simulink model "q4conversor"  (R2023b)
settings: Solver=VariableStepAuto  StartTime=0.0  StopTime=4e-3  RelTol=1e-3
values from neighbouring files (symbols this model uses):
  C = 100e-6    (= 0.0001)    [q4.m]
  Gatr = zpk(Gatr)    [q4.m]
  Gavan = zpk(Gavan)    [q4.m]
  Kc = 198    [q4.m]
  Kd = npid(1)    [q4.m]
  Ki = npid(3)    [q4.m]
  Kp = npid(2)    [q4.m]
  L = 100e-6    (= 0.0001)    [q4.m]
  Rc = 0.5    [q4.m]
  Ro = Vo^2/Po    (= 10)    [q4.m]
libraries: spsSeriesRLCBranchLib x3, cstblocks x2, spsCurrentMeasurementLib x1, spsDiodeLib x1, spsMosfetLib x1, spsPWMGeneratorDCDCLib x1, spsDCVoltageSourceLib x1, spsVoltageMeasurementLib x1, sps_lib x1
settings Model: Creator=aluno-2  LastModifiedBy=aluno-2

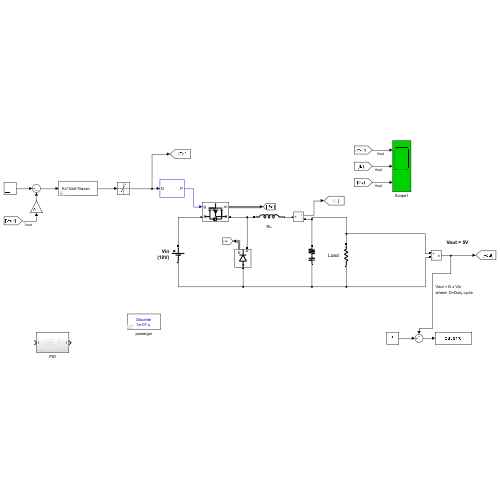
[thumbnail: Simulink's stored preview of the top-level diagram]
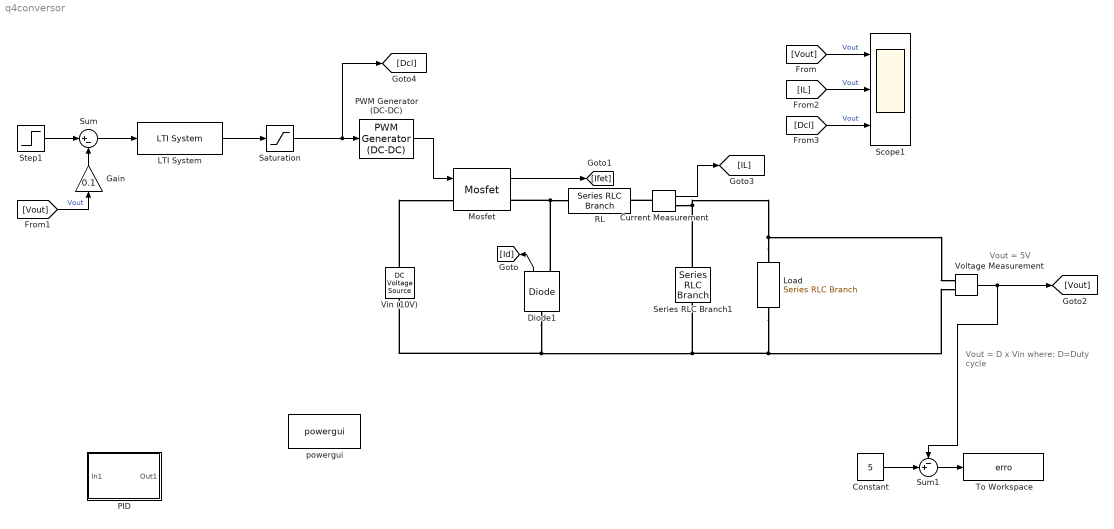
== system q4conversor ==
  note: Vout = D x Vin
      | where: D=Duty cycle
  note: Vout = 5V
  Constant : Constant  Value=5
  Current Measurement : spsCurrentMeasurementLib/Current Measurement  PhasorSimulation=off  OutputType=Complex  PSBequivalent=0
  Diode1 : spsDiodeLib/Diode  Ron=1e-3  Lon=0  Vf=0  IC=0  UseSnubber=off  Rs=inf  Cs=inf  Measurements=on
  Gain : Gain  Gain=0.1
  LTI System : cstblocks/LTI System  sys=Kc*Gatr*Gavan  IC=[]  PadeOrder=0
  Load : spsSeriesRLCBranchLib/Series RLC Branch  LConnTagsString=__new0  RConnTagsString=__new0  BranchType=R  Resistance=Ro  Inductance=200e-6  SetiL0=off  InitialCurrent=0  Capacitance=400e-6  Setx0=off  InitialVoltage=0  Measurements=None
  Mosfet : spsMosfetLib/Mosfet  Ron=1e-3  Lon=0  Rd=1e-3  Vfd=0  IC=0  Rs=1e-3  Cs=100e-9  Measurements=on
  PID : Subsystem
  PWM Generator (DC-DC) : spsPWMGeneratorDCDCLib/PWM Generator (DC-DC)  Fsw=100e3  Ts=0
  RL : spsSeriesRLCBranchLib/Series RLC Branch  LConnTagsString=__new0  RConnTagsString=__new0  BranchType=L  Resistance=0.02  Inductance=L  SetiL0=on  InitialCurrent=2.5/10  Capacitance=1e-6  Setx0=off  InitialVoltage=0  Measurements=None
  Saturation : Saturate  UpperLimit=1  LowerLimit=0
  Scope1 : Scope  NumInputPorts=3
  Series RLC Branch1 : spsSeriesRLCBranchLib/Series RLC Branch  LConnTagsString=__new0  RConnTagsString=__new0  BranchType=RC  Resistance=Rc  Inductance=200e-6  SetiL0=off  InitialCurrent=0  Capacitance=C  Setx0=on  InitialVoltage=5  Measurements=None
  Step1 : Step  Time=0  Before=0.5  After=0.5  SampleTime=0
  Sum : Sum  Inputs=|+-
  Sum1 : Sum  Inputs=-+|
  To Workspace : ToWorkspace  VariableName=erro  SampleTime=-1
  Vin (10V) : spsDCVoltageSourceLib/DC Voltage Source  Amplitude=10  Measurements=None
  Voltage Measurement : spsVoltageMeasurementLib/Voltage Measurement  PhasorSimulation=off  OutputType=Complex  PSBequivalent=0
  powergui : sps_lib/powergui  Priority=1  SimulationMode=Discrete  SampleTime=100e-9  frequency=60  Iterations=50  frequencyindice=0  Pbase=100e6  ErrMax=1e-4  UnitsV=kV  UnitsW=MW  buscounter=0  FunctionMessages=off  echomessages=off  EnableUseOfTLC=off  CurrentSourceSwitches=off  DisableSnubberDevices=off  DisableRonSwitches=off  DisableVfSwitches=off  DisplayEquations=off  AutomaticDiscreteSolvers=off  SolverType=Tustin/Backward Euler (TBE)  Interpol=off  ExternalGateDelay=off  methode=off  Ts=100  x0status=blocks  SPID=on  SwTol=0  HookPort=off  NonlinearTolerance=1e-4  nMaxIteration=100  ContinueOnMaxIteration=on  RestoreLinks=warning  ResistiveCurrentMeasurement=off  Frange=[0:2:500]  Ylog=off  Xlog=on  ShowGrid=off  save=off  variable=ZData  structure=0  ZoomFFT=off  StartTime=0.0  cycles=1  DisplayStyle=1  fundamental=60  FreqAxis=off  MaxFrequency=1000  frequencyindicesteady=1  RmsSteady=1  display=off
  wires:
  Mosfet/1 -> [Ifet]
  [Vout] -> Scope1/1  "Vout"
  Voltage Measurement/1 -> Sum1/1, [Vout]
  PWM Generator (DC-DC)/1 -> Mosfet/1
  Diode1/1 -> [Id]
  Step1/1 -> Sum/1
  Sum/1 -> LTI System/1
  [Vout] -> Gain/1  "Vout"
  Current Measurement/1 -> [IL]
  [IL] -> Scope1/2  "Vout"
  [Dcl] -> Scope1/3  "Vout"
  Gain/1 -> Sum/2
  LTI System/1 -> Saturation/1
  Saturation/1 -> [Dcl], PWM Generator (DC-DC)/1
  Constant/1 -> Sum1/2
  Sum1/1 -> To Workspace/1
  connections:
  Voltage Measurement/LConn2 -- Load/RConn1 -- Vin (10V)/LConn1 -- Diode1/LConn1 -- Series RLC Branch1/RConn1
  Mosfet/RConn1 -- Diode1/RConn1 -- RL/LConn1
  Load/LConn1 -- Current Measurement/RConn1 -- Series RLC Branch1/LConn1 -- Voltage Measurement/LConn1
  Vin (10V)/RConn1 -- Mosfet/LConn1
  Current Measurement/LConn1 -- RL/RConn1

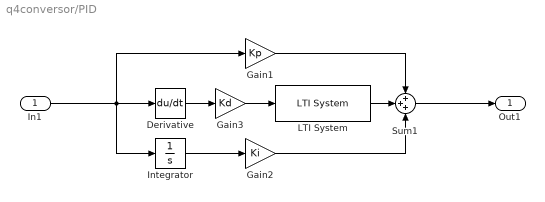
== system q4conversor/PID ==
  In1 : Inport
  Derivative : Derivative
  Gain1 : Gain  Gain=Kp
  Gain2 : Gain  Gain=Ki
  Gain3 : Gain  Gain=Kd
  Integrator : Integrator
  LTI System : cstblocks/LTI System  sys=tf(1,[0.002 1])  IC=[]  PadeOrder=0
  Sum1 : Sum  Inputs=+++
  Out1 : Outport
  wires:
  Gain2/1 -> Sum1/3
  Gain3/1 -> LTI System/1
  In1/1 -> Gain1/1, Integrator/1, Derivative/1
  Derivative/1 -> Gain3/1
  Integrator/1 -> Gain2/1
  Gain1/1 -> Sum1/1
  Sum1/1 -> Out1/1
  LTI System/1 -> Sum1/2
